simulink model "LAB2"  (R2023a)
settings: Solver=VariableStepAuto  StartTime=0.0  StopTime=10.0  RelTol=1e-3
settings Model: Creator=Verbo  LastModifiedBy=sonno

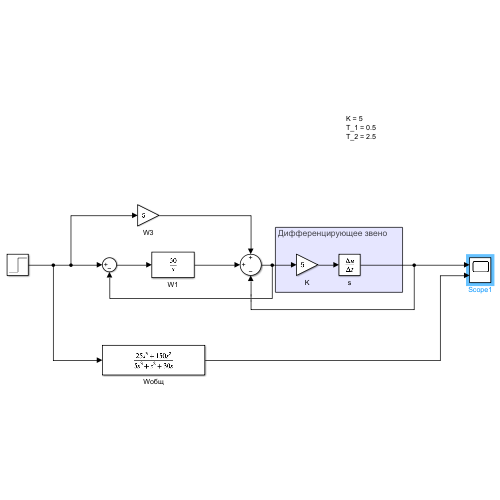
[thumbnail: Simulink's stored preview of the top-level diagram]
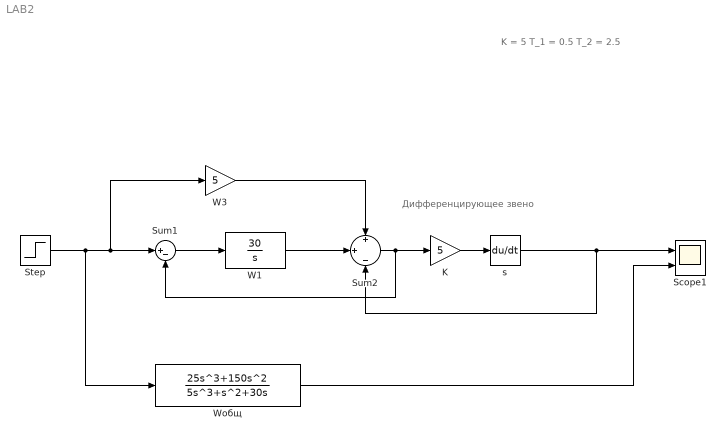
== system LAB2 ==
  note: K = 5
      | T_1 = 0.5
      | T_2 = 2.5
  note: Дифференцирующее звено
  K : Gain  Gain=5
  Scope1 : Scope  NumInputPorts=2
  Step : Step  SampleTime=0
  Sum1 : Sum  Inputs=|+-
  Sum2 : Sum  Inputs=+|+|-
  W1 : TransferFcn  Numerator=[30]  Denominator=[1 0]
  W3 : Gain  Gain=5
  Wобщ : TransferFcn  Numerator=[25 150 0 0]  Denominator=[5 1 30 0]
  s : Derivative  CoefficientInTFapproximation=0
  wires:
  K/1 -> s/1
  Step/1 -> Wобщ/1, W3/1, Sum1/1
  Sum1/1 -> W1/1
  W3/1 -> Sum2/1
  W1/1 -> Sum2/2
  s/1 -> Sum2/3, Scope1/1
  Sum2/1 -> Sum1/2, K/1
  Wобщ/1 -> Scope1/2
